simulink model "sim"  (R2021a)
settings: Solver=ode23tb  StartTime=0.0  StopTime=0.1  MaxStep=5e-6  RelTol=1e-3  EnableMultiTasking=on
libraries: spsDiodeLib x4, spsIGBTDiodeLib x4, spsIGBTLib x4, spsDCVoltageSourceLib x4, spsSeriesRLCBranchLib x1, powerlib_extras x1, spsVoltageMeasurementLib x1, spspowerguiLib x1
settings Model: Creator=kAnnanvalar  LastModifiedBy=madha
settings SolverCC: AlgebraicLoopSolver=TrustRegion
settings DataIOCC: LimitDataPoints=on  SaveFormat=Array  SignalLoggingSaveFormat=ModelDataLogs  ReturnWorkspaceOutputs=off
settings OptimizationCC: ExpressionDepthLimit=2147483647  LifeSpan=inf
settings DebuggingCC: UnderspecifiedInitializationDetection=Classic  MergeDetectMultiDrivingBlocksExec=none  SolverPrmCheckMsg=warning  FcnCallInpInsideContextMsg=warning  StateNameClashWarn=warning  SFUnexpectedBacktrackingDiag=warning  SFNoUnconditionalDefaultTransitionDiag=warning  SFExecutionAtInitializationDiag=none  SFMachineParentedDataDiag=warning  ArithmeticOperatorsInVariantConditions=warning
settings HardwareCC: ProdBitPerPointer=32  ProdBitPerSizeT=32  ProdBitPerPtrDiffT=32  ProdLargestAtomicFloat=None  ProdIntDivRoundTo=Undefined  ProdEndianess=Unspecified  ProdWordSize=32  ProdHWDeviceType=32-bit Generic
settings ModelReferenceCC: PropagateSignalLabelsOutOfModel=off
settings SFSimCC: SimUseLocalCustomCode=off  CustomCodeUndefinedFunction=UseInterfaceOnly
settings RTWCC: RTWUseLocalCustomCode=off
settings CodeAppCC: StateflowObjectComments=on
settings GRTTargetCC: TargetLangStandard=C89/C90 (ANSI)  CodeReplacementLibrary=NOT IN USE  CombineOutputUpdateFcns=off  GRTInterface=on
settings ConfigComp: CovMetricSettings=dw  CovSaveCumulativeToWorkspaceVar=on  CovSaveSingleToWorkspaceVar=on  CovExternalEMLEnable=off
settings SimscapeCC: SimscapeNormalizeSystem=off

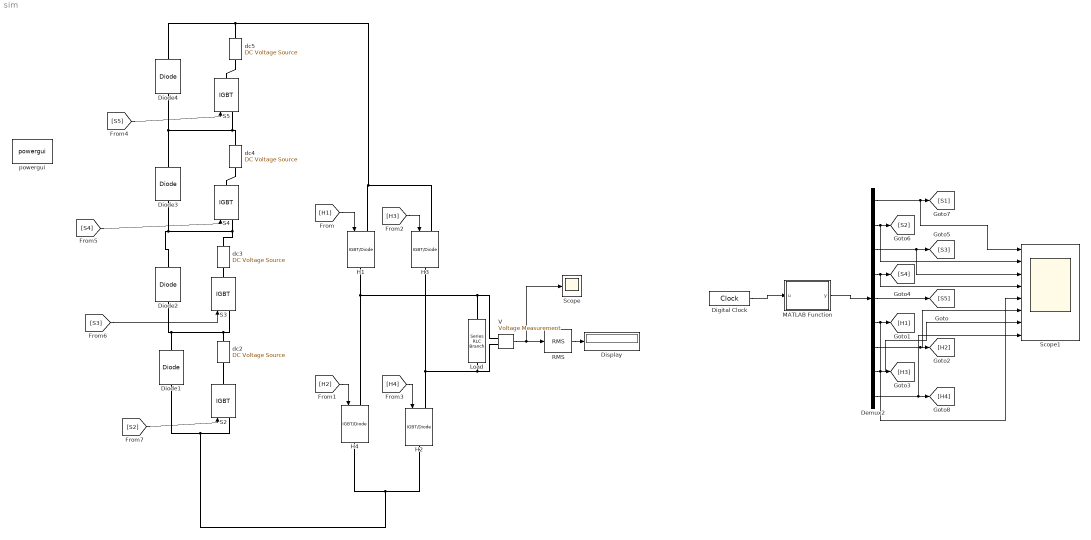
== system sim ==
  Demux2 : Demux  Outputs=9
  Digital Clock : DigitalClock  SampleTime=0.0001
  Diode{1..4} (4 alike) : spsDiodeLib/Diode  Ron=0.001  Lon=0  Vf=0.8  IC=0  UseSnubber=off  Rs=500  Cs=250e-9  Measurements=off
  Display : Display
  H{1..4} (4 alike) : spsIGBTDiodeLib/IGBT//Diode  Ron=1e-3  Rs=1e5  Cs=inf  Measurements=off
  Load : spsSeriesRLCBranchLib/Series RLC Branch  LConnTagsString=__new0  RConnTagsString=__new0  BranchType=R  Resistance=100  Inductance=1e-3  SetiL0=off  InitialCurrent=0  Capacitance=1e-6  Setx0=off  InitialVoltage=0  Measurements=None
  MATLAB Function : MATLAB Function  TreatAsAtomicUnit=on
  RMS : powerlib_extras/Measurements/RMS  f1=50
      settings: SourceProductBaseCode=PS
  S{2..5} (4 alike) : spsIGBTLib/IGBT  Ron=0.001  Lon=0  Vf=1  Tf=1e-6  Tt=2e-6  IC=0  Rs=1e5  Cs=inf  Measurements=off
  Scope : Scope
  Scope1 : Scope  NumInputPorts=8
  V : spsVoltageMeasurementLib/Voltage Measurement  PhasorSimulation=off  OutputType=Complex  PSBequivalent=0
  dc2 : spsDCVoltageSourceLib/DC Voltage Source  Amplitude=12  Measurements=None
  dc3 : spsDCVoltageSourceLib/DC Voltage Source  Amplitude=24  Measurements=None
  dc4 : spsDCVoltageSourceLib/DC Voltage Source  Amplitude=48  Measurements=None
  dc5 : spsDCVoltageSourceLib/DC Voltage Source  Amplitude=96  Measurements=None
  powergui : spspowerguiLib/powergui  Priority=1  SimulationMode=Continuous  SampleTime=50e-6  frequency=60  Iterations=50  frequencyindice=0  Pbase=100e6  ErrMax=1e-4  UnitsV=kV  UnitsW=MW  buscounter=0  FunctionMessages=off  echomessages=off  EnableUseOfTLC=off  CurrentSourceSwitches=on  DisableSnubberDevices=off  DisableRonSwitches=off  DisableVfSwitches=off  DisplayEquations=off  AutomaticDiscreteSolvers=off  SolverType=Tustin  Interpol=off  ExternalGateDelay=off  methode=off  Ts=0  x0status=blocks  SPID=off  SwTol=0  HookPort=off  NonlinearTolerance=1e-4  nMaxIteration=100  ContinueOnMaxIteration=off  RestoreLinks=warning  ResistiveCurrentMeasurement=off  Frange=[0:2:500]  Ylog=off  Xlog=on  ShowGrid=off  save=off  variable=ZData  structure=ScopeData  ZoomFFT=off  StartTime=0.0  cycles=5  DisplayStyle=1  fundamental=50  FreqAxis=off  MaxFrequency=1000  frequencyindicesteady=1  RmsSteady=1  display=off
  wires:
  V/1 -> RMS/1, Scope/1
  RMS/1 -> Display/1
  Digital Clock/1 -> MATLAB Function/1(u)
  MATLAB Function/1(y) -> Demux2/1
  [H1] -> H1/1
  [H2] -> H4/1
  [H3] -> H3/1
  [H4] -> H2/1
  Demux2/8 -> Scope1/7, [H3]
  Demux2/7 -> Scope1/6, [H2]
  Demux2/6 -> Scope1/5, [H1]
  Demux2/4 -> Scope1/4, [S4]
  Demux2/3 -> Scope1/3, [S3]
  Demux2/2 -> Scope1/2, [S2]
  Demux2/1 -> Scope1/1, [S1]
  [S4] -> S4/1
  [S3] -> S3/1
  [S2] -> S2/1
  Demux2/9 -> Scope1/8, [H4]
  [S5] -> S5/1
  Demux2/5 -> [S5]
  connections:
  H1/RConn1 -- Load/LConn1 -- V/LConn1 -- H4/LConn1
  V/LConn2 -- H2/LConn1 -- H3/RConn1 -- Load/RConn1
  dc5/RConn1 -- Diode4/RConn1 -- H1/LConn1 -- H3/LConn1
  dc2/LConn1 -- S2/RConn1
  S3/RConn1 -- dc3/LConn1
  Diode2/RConn1 -- Diode3/LConn1 -- S4/LConn1 -- dc3/RConn1
  H4/RConn1 -- H2/RConn1 -- Diode1/LConn1 -- S2/LConn1
  S3/LConn1 -- Diode1/RConn1 -- Diode2/LConn1 -- dc2/RConn1
  dc4/LConn1 -- S4/RConn1
  dc4/RConn1 -- S5/LConn1 -- Diode4/LConn1 -- Diode3/RConn1
  dc5/LConn1 -- S5/RConn1

== matlab function sim/MATLAB Function ==
  data: u input; y output
function y = fcn(u)
%#codegen

a = 32766*(sin(2*pi*50*u(1)));
if(a > 807)
    s6=1;
    s7=0;
    s8=0;
    s9=1;
else if(a < -807)
    s6=0;
    s7=1;
    s8=1;
    s9=0;
    else
        s6=0;
        s7=0;
        s8=0;
        s9=0;
    end
end

c= abs(a);

if(c < 1023)
    s1 = 0;
    s2 = 0;
    s3 = 0;
    s4 = 0;
    s5 = 0;
else if(c < 2*1023)
    s1 = 1;
    s2 = 0;
    s3 = 0;
    s4 = 0;
    s5 = 0;
else if(c < 3*1023)
    s1 = 0;
    s2 = 1;
    s3 = 0;
    s4 = 0;
    s5 = 0;
else if(c < 4*1023)
    s1 = 1;
    s2 = 1;
    s3 = 0;
    s4 = 0;
    s5 = 0;
else if(c < 5*1023)
    s1 = 0;
    s2 = 0;
    s3 = 1;
    s4 = 0;
    s5 = 0;
else if(c < 6*1023)
    s1 = 1;
    s2 = 0;
    s3 = 1;
    s4 = 0;
    s5 = 0;
else if(c < 7*1023)
    s1 = 0;
    s2 = 1;
    s3 = 1;
    s4 = 0;
    s5 = 0;
else if(c < 8*1023)
    s1 = 1;
    s2 = 1;
    s3 = 1;
    s4 = 0;
    s5 = 0;
else if(c < 9*1023)
    s1 = 0;
    s2 = 0;
    s3 = 0;
    s4 = 1;
    s5 = 0;
else if(c < 10*1023)
    s1 = 1;
    s2 = 0;
    s3 = 0;
    s4 = 1;
    s5 = 0;
else if(c < 11*1023)
    s1 = 0;
    s2 = 1;
    s3 = 0;
    s4 = 1;
    s5 = 0;
else if(c < 12*1023)
    s1 = 1;
    s2 = 1;
    s3 = 0;
    s4 = 1;
    s5 = 0;
else if(c < 13*1023)
    s1 = 0;
    s2 = 0;
    s3 = 1;
    s4 = 1;
    s5 = 0;
else if(c < 14*1023)
    s1 = 1;
    s2 = 0;
    s3 = 1;
    s4 = 1;
    s5 = 0;
else if(c < 15*1023)
    s1 = 0;
    s2 = 1;
    s3 = 1;
    s4 = 1;
    s5 = 0;
else if(c < 16*1023)
    s1 = 1;
    s2 = 1;
    s3 = 1;
    s4 = 1;
    s5 = 0;
else if(c < 17*1023)
    s1 = 0;
    s2 = 0;
    s3 = 0;
    s4 = 0;
    s5 = 1;
else if(c < 18*1023)
    s1 = 1;
    s2 = 0;
    s3 = 0;
    s4 = 0;
    s5 = 1;
else if(c < 19*1023)
    s1 = 0;
    s2 = 1;
    s3 = 0;
    s4 = 0;
    s5 = 1;
else if(c < 20*1023)
    s1 = 1;
    s2 = 1;
    s3 = 0;
    s4 = 0;
    s5 = 1;
else if(c < 21*1023)
    s1 = 0;
    s2 = 0;
    s3 = 1;
    s4 = 0;
    s5 = 1;
else if(c < 22*1023)
    s1 = 1;
    s2 = 0;
    s3 = 1;
    s4 = 0;
    s5 = 1;
else if(c < 23*1023)
    s1 = 0;
    s2 = 1;
    s3 = 1;
    s4 = 0;
    s5 = 1;
else if(c < 24*1023)
    s1 = 1;
    s2 = 1;
    s3 = 1;
    s4 = 0;
    s5 = 1;
else if(c < 25*1023)
    s1 = 0;
    s2 = 0;
    s3 = 0;
    s4 = 1;
    s5 = 1;
else if(c < 26*1023)
    s1 = 1;
    s2 = 0;
    s3 = 0;
    s4 = 1;
    s5 = 1;
else if(c < 27*1023)
    s1 = 0;
    s2 = 1;
    s3 = 0;
    s4 = 1;
    s5 = 1;
else if(c < 28*1023)
    s1 = 1;
    s2 = 1;
    s3 = 0;
    s4 = 1;
    s5 = 1;
else if(c < 29*1023)
    s1 = 0;
    s2 = 0;
    s3 = 1;
    s4 = 1;
    s5 = 1;
else if(c < 30*1023)
    s1 = 1;
    s2 = 0;
    s3 = 1;
    s4 = 1;
    s5 = 1;
else if(c < 31*1023)
    s1 = 0;
    s2 = 1;
    s3 = 1;
    s4 = 1;
    s5 = 1;
else if(c > 31*1023)
    s1 = 1;
    s2 = 1;
    s3 = 1;
    s4 = 1;
    s5 = 1;
    else
        s1=0;
        s2=0;
        s3=0;
        s4=0;
        s5=0;
   end
   end
  end
   end
   end
   end
   end
    end
    end
    end
    end
    end
    end
    end
    end
    end
    end
    end
    end
    end
    end
    end
    end
    end
    end
    end
    end
    end
    end
    end
    end
end

y = [s1,s2,s3,s4,s5,s6,s7,s8,s9];

end
